simulink model "Lab2_Second_Order"  (R2024b)
settings: Solver=VariableStepAuto  StartTime=0.0  StopTime=10.0  RelTol=1e-3
settings Model: Creator=Ahmad  LastModifiedBy=Ahmad

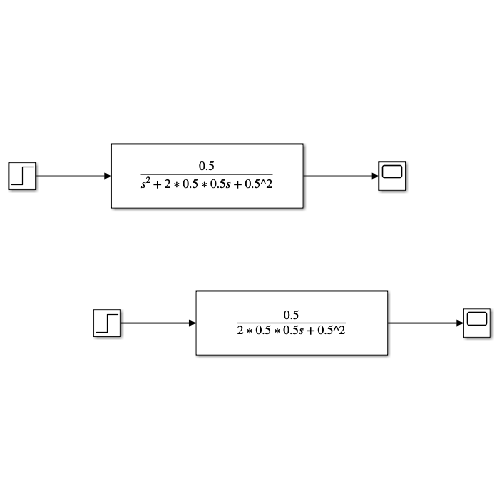
[thumbnail: Simulink's stored preview of the top-level diagram]
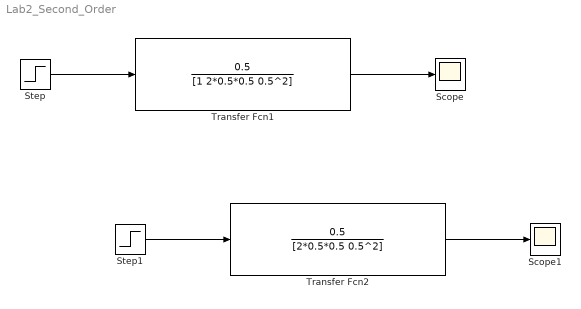
== system Lab2_Second_Order ==
  Scope : Scope
  Scope1 : Scope
  Step : Step  SampleTime=0
  Step1 : Step  SampleTime=0
  Transfer Fcn1 : TransferFcn  Numerator=[0 0.5]  Denominator=[1 2*0.5*0.5 0.5^2]
  Transfer Fcn2 : TransferFcn  Numerator=[0 0.5]  Denominator=[2*0.5*0.5 0.5^2]
  wires:
  Step/1 -> Transfer Fcn1/1
  Transfer Fcn1/1 -> Scope/1
  Step1/1 -> Transfer Fcn2/1
  Transfer Fcn2/1 -> Scope1/1
